simulink model "Problema_2_simulink"  (R2014a)
settings: Solver=ode15s  StartTime=0.0  StopTime=15  RelTol=1e-3
values from neighbouring files (symbols this model uses):
  b = 0.5    [Problema_2_tp2_variables.m]
  g = 9.8    [Problema_2_tp2_variables.m]
  k = 2    [Problema_2_tp2_variables.m]
  L = 0.01    [Problema_2_tp2_variables.m]
  M = 0.2    [Problema_2_tp2_variables.m]
  R = 20    [Problema_2_tp2_variables.m]
settings Model: Creator=lraff  LastModifiedBy=lraff
settings DataIOCC: LimitDataPoints=off  MaxDataPoints=5000

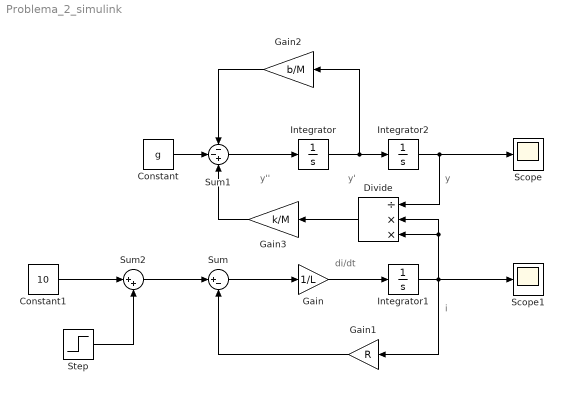
== system Problema_2_simulink ==
  note: di/dt
  note: i
  note: y''
  note: y'
  note: y
  Constant : Constant  Value=g
  Constant1 : Constant  Value=10
  Divide : Product  Inputs=/**
  Gain : Gain  Gain=1/L
  Gain1 : Gain  Gain=R
  Gain2 : Gain  Gain=b/M
  Gain3 : Gain  Gain=k/M
  Integrator : Integrator
  Integrator1 : Integrator
  Integrator2 : Integrator  InitialCondition=0.001
  Scope : Scope
      settings: TimeRange=4.662835249042145  YMin=-0.0976995085332798  YMax=0.5017925786241709
  Scope1 : Scope
  Step : Step  Time=6  After=2  SampleTime=0
  Sum : Sum  Inputs=|+-
  Sum1 : Sum  Inputs=--+
  Sum2 : Sum  Inputs=|++
  wires:
  Sum/1 -> Gain/1
  Gain/1 -> Integrator1/1
  Gain1/1 -> Sum/2
  Integrator1/1 -> Scope1/1, Gain1/1, Divide/2, Divide/3
  Sum1/1 -> Integrator/1
  Integrator/1 -> Gain2/1, Integrator2/1
  Gain2/1 -> Sum1/1
  Integrator2/1 -> Scope/1, Divide/1
  Divide/1 -> Gain3/1
  Gain3/1 -> Sum1/3
  Constant/1 -> Sum1/2
  Constant1/1 -> Sum2/1
  Sum2/1 -> Sum/1
  Step/1 -> Sum2/2
